simulink model "URM_6_test"  (R2014a)
settings: Solver=ode45  StartTime=0.0  StopTime=tmax  RelTol=1e-3
values from neighbouring files (symbols this model uses):
  a1 = 2    [URM_SP.m]
  a2 = 1.5    [URM_SP.m]
  a3 = 0.5    [URM_SP.m]
  uhel_phi = mesh_phi(i)    [URM_SP.m]
  vmax = 1    [URM_SP.m]
settings Model: Creator=Julie  LastModifiedBy=kajak_000
settings SimMechanicsCC: VisOnUpdateDiagram=on  VisDuringSimulation=on

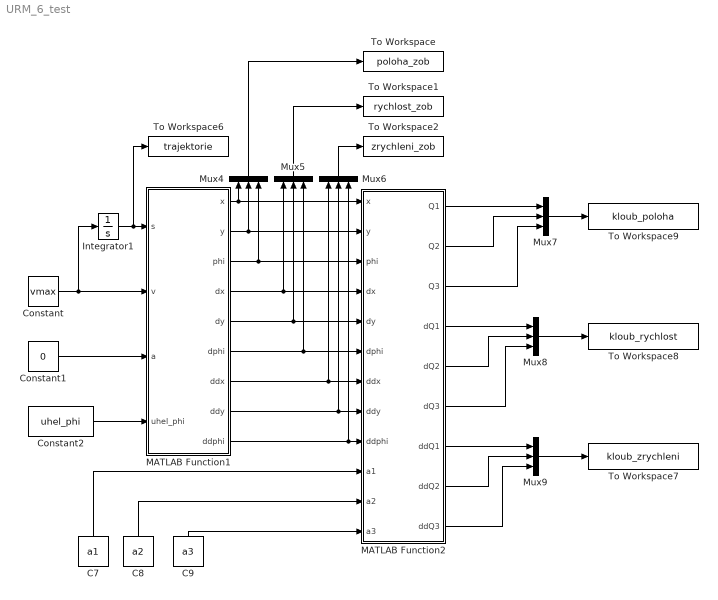
== system URM_6_test ==
  C7 : Constant  Value=a1
  C8 : Constant  Value=a2
  C9 : Constant  Value=a3
  Constant : Constant  Value=vmax
  Constant1 : Constant  Value=0
  Constant2 : Constant  Value=uhel_phi
  Integrator1 : Integrator
  MATLAB Function1 : MATLAB Function  TreatAsAtomicUnit=on
  MATLAB Function2 : MATLAB Function  TreatAsAtomicUnit=on
  Mux{4..9} (6 alike) : Mux  Inputs=3
  To Workspace : ToWorkspace  VariableName=poloha_zob  SaveFormat=Structure With Time  SampleTime=-1
  To Workspace1 : ToWorkspace  VariableName=rychlost_zob  SaveFormat=Structure With Time  SampleTime=-1
  To Workspace2 : ToWorkspace  VariableName=zrychleni_zob  SaveFormat=Structure With Time  SampleTime=-1
  To Workspace6 : ToWorkspace  VariableName=trajektorie  SaveFormat=Structure With Time  SampleTime=-1
  To Workspace7 : ToWorkspace  VariableName=kloub_zrychleni  SaveFormat=Structure With Time  SampleTime=-1
  To Workspace8 : ToWorkspace  VariableName=kloub_rychlost  SaveFormat=Structure With Time  SampleTime=-1
  To Workspace9 : ToWorkspace  VariableName=kloub_poloha  SaveFormat=Structure With Time  SampleTime=-1
  wires:
  C9/1 -> MATLAB Function2/12(a3)
  C8/1 -> MATLAB Function2/11(a2)
  C7/1 -> MATLAB Function2/10(a1)
  MATLAB Function2/1(Q1) -> Mux7/1
  MATLAB Function2/2(Q2) -> Mux7/2
  MATLAB Function2/3(Q3) -> Mux7/3
  MATLAB Function2/4(dQ1) -> Mux8/1
  MATLAB Function2/5(dQ2) -> Mux8/2
  MATLAB Function2/6(dQ3) -> Mux8/3
  MATLAB Function2/9(ddQ3) -> Mux9/3
  MATLAB Function2/8(ddQ2) -> Mux9/2
  MATLAB Function2/7(ddQ1) -> Mux9/1
  Constant/1 -> MATLAB Function1/2(v), Integrator1/1
  Integrator1/1 -> To Workspace6/1, MATLAB Function1/1(s)
  Constant1/1 -> MATLAB Function1/3(a)
  MATLAB Function1/1(x) -> MATLAB Function2/1(x), Mux4/1
  MATLAB Function1/2(y) -> MATLAB Function2/2(y), Mux4/2
  MATLAB Function1/4(dx) -> Mux5/1, MATLAB Function2/4(dx)
  MATLAB Function1/5(dy) -> Mux5/2, MATLAB Function2/5(dy)
  MATLAB Function1/6(dphi) -> Mux5/3, MATLAB Function2/6(dphi)
  MATLAB Function1/7(ddx) -> Mux6/1, MATLAB Function2/7(ddx)
  MATLAB Function1/8(ddy) -> Mux6/2, MATLAB Function2/8(ddy)
  MATLAB Function1/9(ddphi) -> Mux6/3, MATLAB Function2/9(ddphi)
  Mux6/1 -> To Workspace2/1
  Mux5/1 -> To Workspace1/1
  MATLAB Function1/3(phi) -> MATLAB Function2/3(phi), Mux4/3
  Constant2/1 -> MATLAB Function1/4(uhel_phi)
  Mux9/1 -> To Workspace7/1
  Mux8/1 -> To Workspace8/1
  Mux7/1 -> To Workspace9/1
  Mux4/1 -> To Workspace/1

== matlab function URM_6_test/MATLAB Function1 ==
  data: x output; s input; y output; v input; a input; phi output; dx output; dy output; dphi output; ddx output; ddy output; ddphi output; uhel_phi input
function [x, y, phi, dx, dy, dphi, ddx, ddy, ddphi] = fcn(s, v, a, uhel_phi)
%#codegen
% x,y,phi pozadovana poloha + natoceni koncoveho efektoru
% dx,dy,dphi pozadovana rychlost + uhlova rychlost
% ddx,ddy,ddphi pozadovane zrychleni + uhlove zrychleni
%% IOKU trajektorie
A = [2; 0.5]; % bod A
B = [0; 1]; % bod B
C = [2; 2.5]; % bod C
r = 0.3; % polomer kruznice
vmax = 1; % maximalni rychlost
dir = -1;

nBA = (A - B)/ norm(A-B); % smerovy vektor z B do A
nBC = (C - B)/ norm(C-B); % smerovy vektor z B do C
nBS = (nBA  + nBC)/norm(nBA  + nBC); % smerovy vektor z B do S

K1 = nBA * nBA' * nBS - nBS; 
l = r/(sqrt(K1' * K1)); % konstantni vzdalenost z B do S
S = B + nBS * l; % souradnice stredu kruznice
k = nBA' * (A - S); 

PA = A - nBA * k; % pocatecni bod oblouku
PC = B + norm(PA - B) * nBC; %koncovy bod oblouku

dPhi = acos((PC - S)' * (PA - S) / r^2); %delta phi
SPA = (PA - S);
phiPA = atan2(SPA(2), SPA(1));

s1 = norm(PA - A); % prvni usek - usecka
sk = r * dPhi; %druhy usek - oblouk
s2 = norm(PC - C); % treti usek - usecka

smax = s1 + sk + s2; % maximalni draha
tmax = smax/vmax; % maximalni cas

if s >=0 && s < s1
    k1 = s;
    dk1 = v;
    ddk1 = a;
    X = [A - k1*nBA; 0];
    dX = [-dk1 * nBA; 0];
    ddX = [-ddk1 * nBA; 0];
    
elseif s1 <= s && s < s1 + sk
    Phi = (s - s1)/r; % uhel urcujici jak daleko na oblouku jsme (ruzne od phi)
    dPhi = v/r;
    ddPhi = a/r;
    X = [r * [cos(phiPA + dir * Phi); sin(phiPA + dir * Phi)] + S; 0];
    dX = [r * [-sin(phiPA + dir * Phi); cos(phiPA + dir * Phi)] * dir * dPhi; 0];
    ddX = [r * [-cos(phiPA + dir * Phi); -sin(phiPA + dir * Phi)] * dir^2 * dPhi^2 + r * [-sin(phiPA + dir * Phi); cos(phiPA + dir * Phi)] * dir * ddPhi; 0];
        
elseif s1 + sk <= s && s <= s1 + sk + s2
    k2 = s - s1 - sk;
    dk2 = v;
    ddk2 = a;
    X = [PC + k2*nBC; 0];
    dX = [dk2 * nBC; 0];
    ddX = [ddk2 * nBC; 0];
else
    X = [0; 0; 0];
    dX = [0; 0; 0];
    ddX = [0; 0; 0];
end

x = X(1);
y = X(2);
phi = uhel_phi;
dx = dX(1);
dy = dX(2);
dphi = dX(3);
ddx = ddX(1);
ddy = ddX(2);
ddphi = ddX(3);

== matlab function URM_6_test/MATLAB Function2 ==
  data: Q1 output; Q2 output; Q3 output; dQ1 output; dQ2 output; dQ3 output; ddQ1 output; x input; y input; phi input; dx input; dy input; dphi input; ddx input; ddy input; ddphi input; a1 input; a2 input; a3 input; ddQ2 output; ddQ3 output
function [Q1, Q2, Q3, dQ1, dQ2, dQ3, ddQ1, ddQ2, ddQ3] = IOKU(x, y, phi, dx, dy, dphi, ddx, ddy, ddphi, a1, a2, a3)
%% vypocet Q2
cosQ2 = ((x - a3*cos(phi))^2 + (y - a3*sin(phi))^2 - a1^2 - a2^2)/(2 * a1 * a2);
sinQ2 = -abs(sqrt((1 - cosQ2^2))); %jeste zkontrolovat meze u slider gainu
Q2 = atan2(sinQ2, cosQ2);
%% vypocet Q1
A = [-a2 * sinQ2, a2 * cosQ2 + a1; a2 * cosQ2 + a1, a2 * sinQ2];
B = [x - a3*cos(phi); y - a3*sin(phi)];
v = A\B;
sinQ1 = v(1);
cosQ1 = v(2);
Q1 = atan2(sinQ1, cosQ1);
%% vypocet Q3
Q3 = phi - Q1 - Q2;
% rychlost dX
jQ = [-a3 * sin(Q1 + Q2 + Q3) - a2 * sin(Q1 + Q2) - a1 * sin(Q1), -a3 * sin(Q1 + Q2 + Q3) - a2 * sin(Q1 + Q2), -a3 * sin(Q1 + Q2 + Q3);...
    a3 * cos(Q1 + Q2 + Q3) + a2 * cos(Q1 + Q2) + a1 * cos(Q1), a3 * cos(Q1 + Q2 + Q3) + a2 * cos(Q1 + Q2), a3 * cos(Q1 + Q2 + Q3);...
    1, 1, 1];
dX = [dx; dy; dphi];
dQ = jQ^-1 * dX;
dQ1 = dQ(1);
dQ2 = dQ(2);
dQ3 = dQ(3);

% zrychleni ddX
djQ = [-a3*cos(Q1+Q2+Q3)*(dQ1+dQ2+dQ3) - a2*cos(Q1+Q2)*(dQ1+dQ2) - a1*cos(Q1)*dQ1, -a3*cos(Q1+Q2+Q3)*(dQ1+dQ2+dQ3) - a2*cos(Q1+Q2)*(dQ1+dQ2), -a3*cos(Q1+Q2+Q3)*(dQ1+dQ2+dQ3);...
    -a3*sin(Q1+Q2+Q3)*(dQ1+dQ2+dQ3) - a2*sin(Q1+Q2)*(dQ1+dQ2) - a1*sin(Q1)*dQ1, -a3*sin(Q1+Q2+Q3)*(dQ1+dQ2+dQ3) - a2*sin(Q1+Q2)*(dQ1+dQ2), -a3*sin(Q1+Q2+Q3)*(dQ1+dQ2+dQ3);...
    0, 0, 0];
ddX = [ddx; ddy; ddphi];
ddQ = jQ^-1 * (ddX - djQ * dQ);
ddQ1 = ddQ(1);
ddQ2 = ddQ(2);
ddQ3 = ddQ(3);
